simulink model "TVC_Rocket"  (R2026a)
settings: Solver=VariableStepAuto  StopTime=120
values from neighbouring files (symbols this model uses):
  Iyy = 0.0153455729167    [TVC_results_baseline.mat]
  Kp = 5    [TVC_results_baseline.mat]
  L = 0.55    [TVC_results_baseline.mat]
  servo_max = 15    [TVC_results_baseline.mat]
  servo_min = -15    [TVC_results_baseline.mat]
libraries: slpidlib x2
settings Model: Creator=haquangchuong  LastModifiedBy=haquangchuong

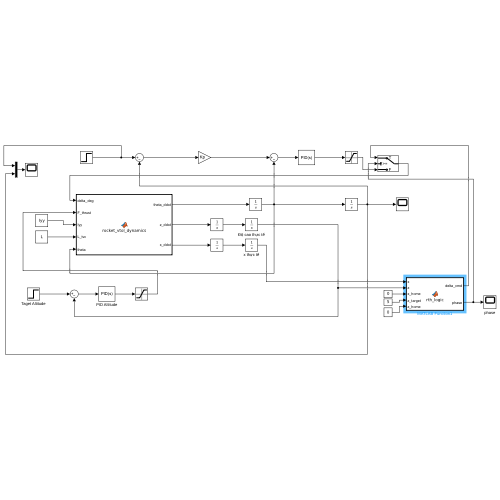
[thumbnail: Simulink's stored preview of the top-level diagram]
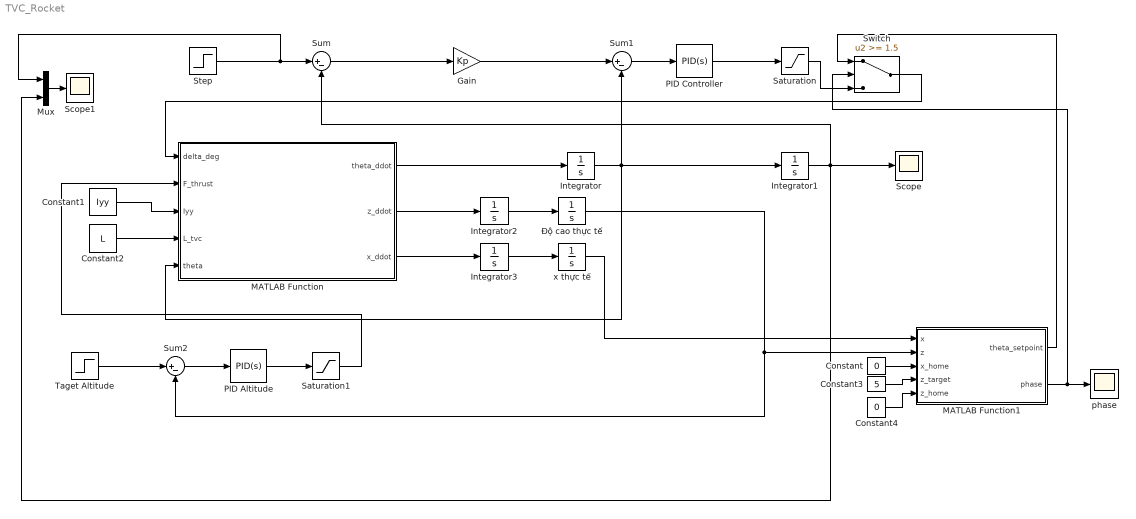
== system TVC_Rocket ==
  Constant : Constant  Value=0
  Constant1 : Constant  Value=Iyy
  Constant2 : Constant  Value=L
  Constant3 : Constant  Value=5
  Constant4 : Constant  Value=0
  Gain : Gain  Gain=Kp
  Integrator{,1..3} (4 alike) : Integrator
  MATLAB Function : MATLAB Function  TreatAsAtomicUnit=on
  MATLAB Function1 : MATLAB Function  TreatAsAtomicUnit=on
  Mux : Mux  Inputs=2
  PID Altitude : slpidlib/PID Controller  Controller=PID  Form=Parallel  TimeDomain=Continuous-time  UseExternalTs=off  SampleTime=-1  IntegratorMethod=Forward Euler  FilterMethod=Forward Euler  ControllerParametersSource=internal  P=2.0  I=0.005  UseKiTs=off  D=1.0  UseExternalDerivativeSource=off  N=100  UseFilter=on  TunerSelectOption=Transfer Function Based (PID Tuner App)  InitialConditionSource=internal  InitialConditionForIntegrator=0  InitialConditionForFilter=0  DifferentiatorICPrevScaledInput=0  ExternalReset=none  TrackingMode=off  Kt=1  LimitOutput=off  SatLimitsSource=internal  UpperSaturationLimit=inf  LowerSaturationLimit=-inf  LinearizeAsGain=on  AntiWindupMode=none  Kb=1  LimitIntegrator=off  UpperIntegratorSaturationLimit=inf  LowerIntegratorSaturationLimit=-inf  POutMin=[]  POutMax=[]  IOutMin=[]  IOutMax=[]  DOutMin=[]  DOutMax=[]  NOutMin=[]  NOutMax=[]  SumOutMin=[]  SumOutMax=[]  SaturationOutMin=[]  SaturationOutMax=[]  PParamMin=[]  PParamMax=[]  IParamMin=[]  IParamMax=[]  DParamMin=[]  DParamMax=[]  NParamMin=[]  NParamMax=[]  KbParamMin=[]  KbParamMax=[]  KtParamMin=[]  KtParamMax=[]  KbOutMin=[]  KbOutMax=[]  KtOutMin=[]  KtOutMax=[]  IntegratorOutMin=[]  IntegratorOutMax=[]  FilterOutMin=[]  FilterOutMax=[]  SumI1OutMin=[]  SumI1OutMax=[]  SumI2OutMin=[]  SumI2OutMax=[]  SumI3OutMin=[]  SumI3OutMax=[]  SumI4OutMin=[]  SumI4OutMax=[]  SumDOutMin=[]  SumDOutMax=[]  DifferentiatorOutMin=[]  DifferentiatorOutMax=[]  FilterDiffOutCoefMin=[]  FilterDiffOutCoefMax=[]  ReciprocalOutMin=[]  ReciprocalOutMax=[]  SumDenOutMin=[]  SumDenOutMax=[]  SumNumOutMin=[]  SumNumOutMax=[]  DivideOutMin=[]  DivideOutMax=[]  UdiffTsProdOutMin=[]  UdiffTsProdOutMax=[]  NTsProdOutMin=[]  NTsProdOutMax=[]  UintegralTsProdOutMin=[]  UintegralTsProdOutMax=[]  UngainTsProdOutMin=[]  UngainTsProdOutMax=[]  ClampingZeroOutDataTypeStr=Inherit: Inherit via back propagation  ClampingZeroOutMin=[]  ClampingZeroOutMax=[]  FilterDenConstantOutDataTypeStr=Inherit: Inherit via back propagation  FilterDenConstantOutMin=[]  FilterDenConstantOutMax=[]  PCopyOutDataTypeStr=Inherit: Inherit via back propagation  PCopyOutMin=[]  PCopyOutMax=[]  NCopyOutDataTypeStr=Inherit: Inherit via back propagation  NCopyOutMin=[]  NCopyOutMax=[]  IntegratorContinuousStateAttributes=''  IntegratorStateMustResolveToSignalObject=off  IntegratorRTWStateStorageClass=Auto  FilterContinuousStateAttributes=''  FilterStateMustResolveToSignalObject=off  FilterRTWStateStorageClass=Auto  ParallelPVariant=InternalParameters  IdealPVariant=Disabled  IVariant=InternalParameters  DVariant=InternalParameters  IntegratorVariant=Continuous  SatVariant=Disabled  AWVariant=Passthrough  PCopyVariant=Disabled  TRVariant=Disabled  FdbkBlocksVariant=Forward  IdealPFdbkVariant=Disabled  SatFdbkVariant=Disabled  DerivativeFilterVariant=ContFilter  NVariant=InternalParameters  NCopyVariant=Disabled  FilterICVariant=InternalICsFilter  IntegratorICVariant=InternalICs  ExternalResetVariant=Disabled  TRSumVariant=Passthrough  SumFdbkVariant=Disabled  SumVariant=Sum_PID  TsampFilterVariant=InternalTs  TsampNgainVariant=Passthrough  TsampIntegralVariant=Disabled_SignalSpec  ExternalSaturationOutDataTypeStr=Inherit: Same as second input  DerivativeSourceVariant=ErrorSignal  PreIntVariant=InternalPreInt
  PID Controller : slpidlib/PID Controller  Controller=PID  Form=Parallel  TimeDomain=Continuous-time  UseExternalTs=off  SampleTime=-1  IntegratorMethod=Forward Euler  FilterMethod=Forward Euler  ControllerParametersSource=internal  P=1.5  I=0.01  UseKiTs=off  D=0.8  UseExternalDerivativeSource=off  N=100  UseFilter=on  TunerSelectOption=Transfer Function Based (PID Tuner App)  InitialConditionSource=internal  InitialConditionForIntegrator=0  InitialConditionForFilter=0  DifferentiatorICPrevScaledInput=0  ExternalReset=none  TrackingMode=off  Kt=1  LimitOutput=off  SatLimitsSource=internal  UpperSaturationLimit=inf  LowerSaturationLimit=-inf  LinearizeAsGain=on  AntiWindupMode=none  Kb=1  LimitIntegrator=off  UpperIntegratorSaturationLimit=inf  LowerIntegratorSaturationLimit=-inf  POutMin=[]  POutMax=[]  IOutMin=[]  IOutMax=[]  DOutMin=[]  DOutMax=[]  NOutMin=[]  NOutMax=[]  SumOutMin=[]  SumOutMax=[]  SaturationOutMin=[]  SaturationOutMax=[]  PParamMin=[]  PParamMax=[]  IParamMin=[]  IParamMax=[]  DParamMin=[]  DParamMax=[]  NParamMin=[]  NParamMax=[]  KbParamMin=[]  KbParamMax=[]  KtParamMin=[]  KtParamMax=[]  KbOutMin=[]  KbOutMax=[]  KtOutMin=[]  KtOutMax=[]  IntegratorOutMin=[]  IntegratorOutMax=[]  FilterOutMin=[]  FilterOutMax=[]  SumI1OutMin=[]  SumI1OutMax=[]  SumI2OutMin=[]  SumI2OutMax=[]  SumI3OutMin=[]  SumI3OutMax=[]  SumI4OutMin=[]  SumI4OutMax=[]  SumDOutMin=[]  SumDOutMax=[]  DifferentiatorOutMin=[]  DifferentiatorOutMax=[]  FilterDiffOutCoefMin=[]  FilterDiffOutCoefMax=[]  ReciprocalOutMin=[]  ReciprocalOutMax=[]  SumDenOutMin=[]  SumDenOutMax=[]  SumNumOutMin=[]  SumNumOutMax=[]  DivideOutMin=[]  DivideOutMax=[]  UdiffTsProdOutMin=[]  UdiffTsProdOutMax=[]  NTsProdOutMin=[]  NTsProdOutMax=[]  UintegralTsProdOutMin=[]  UintegralTsProdOutMax=[]  UngainTsProdOutMin=[]  UngainTsProdOutMax=[]  ClampingZeroOutDataTypeStr=Inherit: Inherit via back propagation  ClampingZeroOutMin=[]  ClampingZeroOutMax=[]  FilterDenConstantOutDataTypeStr=Inherit: Inherit via back propagation  FilterDenConstantOutMin=[]  FilterDenConstantOutMax=[]  PCopyOutDataTypeStr=Inherit: Inherit via back propagation  PCopyOutMin=[]  PCopyOutMax=[]  NCopyOutDataTypeStr=Inherit: Inherit via back propagation  NCopyOutMin=[]  NCopyOutMax=[]  IntegratorContinuousStateAttributes=''  IntegratorStateMustResolveToSignalObject=off  IntegratorRTWStateStorageClass=Auto  FilterContinuousStateAttributes=''  FilterStateMustResolveToSignalObject=off  FilterRTWStateStorageClass=Auto  ParallelPVariant=InternalParameters  IdealPVariant=Disabled  IVariant=InternalParameters  DVariant=InternalParameters  IntegratorVariant=Continuous  SatVariant=Disabled  AWVariant=Passthrough  PCopyVariant=Disabled  TRVariant=Disabled  FdbkBlocksVariant=Forward  IdealPFdbkVariant=Disabled  SatFdbkVariant=Disabled  DerivativeFilterVariant=ContFilter  NVariant=InternalParameters  NCopyVariant=Disabled  FilterICVariant=InternalICsFilter  IntegratorICVariant=InternalICs  ExternalResetVariant=Disabled  TRSumVariant=Passthrough  SumFdbkVariant=Disabled  SumVariant=Sum_PID  TsampFilterVariant=InternalTs  TsampNgainVariant=Passthrough  TsampIntegralVariant=Disabled_SignalSpec  ExternalSaturationOutDataTypeStr=Inherit: Same as second input  DerivativeSourceVariant=ErrorSignal  PreIntVariant=InternalPreInt
  Saturation : Saturate  UpperLimit=servo_max  LowerLimit=servo_min
  Saturation1 : Saturate
  Scope : Scope
      settings: ActiveDisplayYMinimum=-17.498185501340227  ActiveDisplayYMaximum=33.688920146330474
  Scope1 : Scope
      settings: ActiveDisplayYMinimum=-24.629671533739579  ActiveDisplayYMaximum=40.871041025678686
  Step : Step  FinalValue=5  SampleTime=0
  Sum : Sum  Inputs=|+-
  Sum1 : Sum  Inputs=|+-
  Sum2 : Sum  Inputs=|+-
  Switch : Switch  Threshold=1.5  SaturateOnIntegerOverflow=off  InputSameDT=off
  Taget Altitude : Step  FinalValue=5  SampleTime=0
  phase : Scope
      settings: ActiveDisplayYMinimum=1.2513737905524991  ActiveDisplayYMaximum=3.346104044701578  DataLoggingVariableName=ScopeData2
  x thực tế : Integrator
  Độ cao thực tế : Integrator
  wires:
  MATLAB Function/1(theta_ddot) -> Integrator/1
  Integrator/1 -> MATLAB Function/5(theta), Integrator1/1, Sum1/2
  Constant1/1 -> MATLAB Function/3(Iyy)
  Constant2/1 -> MATLAB Function/4(L_tvc)
  Step/1 -> Mux/1, Sum/1
  Integrator1/1 -> Mux/2, Scope/1, Sum/2
  Sum/1 -> Gain/1
  Gain/1 -> Sum1/1
  Sum1/1 -> PID Controller/1
  PID Controller/1 -> Saturation/1
  Mux/1 -> Scope1/1
  MATLAB Function/2(z_ddot) -> Integrator2/1
  Integrator2/1 -> Độ cao thực tế/1
  Taget Altitude/1 -> Sum2/1
  Độ cao thực tế/1 -> MATLAB Function1/2(z), Sum2/2
  Sum2/1 -> PID Altitude/1
  PID Altitude/1 -> Saturation1/1
  Saturation1/1 -> MATLAB Function/2(F_thrust)
  MATLAB Function/3(x_ddot) -> Integrator3/1
  Integrator3/1 -> x thực tế/1
  Constant/1 -> MATLAB Function1/3(x_home)
  Constant3/1 -> MATLAB Function1/4(z_target)
  Constant4/1 -> MATLAB Function1/5(z_home)
  x thực tế/1 -> MATLAB Function1/1(x)
  MATLAB Function1/2(phase) -> phase/1, Switch/2
  Switch/1 -> MATLAB Function/1(delta_deg)
  Saturation/1 -> Switch/3
  MATLAB Function1/1(theta_setpoint) -> Switch/1

== matlab function TVC_Rocket/MATLAB Function1 ==
  data: x input; theta_setpoint output; z input; x_home input; z_target input; z_home input; phase output
function [theta_setpoint, phase] = rth_logic(x, z, x_home, z_target, z_home)
    altitude = -z;
    x_error = x_home - x;

    if altitude < z_target - 0.5
        phase = 1;
        theta_setpoint = 0;

    elseif abs(x_error) > 0.3
        phase = 2;
        % Nghiêng nhẹ để bay ngang — max 3 độ
        theta_setpoint = max(min(0.5 * x_error, 3), -3);

    elseif altitude > 0.1
        phase = 3;
        theta_setpoint = 0;

    else
        phase = 4;
        theta_setpoint = 0;
    end
end

== matlab function TVC_Rocket/MATLAB Function ==
  data: delta_deg input; theta_ddot output; F_thrust input; Iyy input; L_tvc input; theta input; z_ddot output; x_ddot output
function [theta_ddot, z_ddot, x_ddot] = rocket_vtol_dynamics(delta_deg, F_thrust, Iyy, L_tvc, theta)
    m = 0.605;
    g = 9.81;
    delta_rad = deg2rad(delta_deg);
    theta_rad = deg2rad(theta);

    % Trục Pitch
    torque = F_thrust * sin(delta_rad) * L_tvc ...
           - m * g * (L_tvc * 0.5) * sin(theta_rad);
    theta_ddot = torque / Iyy;

    % Trục Z (Cao độ)
    F_vertical = F_thrust * cos(delta_rad + theta_rad);
    z_ddot = (F_vertical - m*g) / m;

    % Trục X (Ngang — RTH cần cái này)
    F_horizontal = F_thrust * sin(delta_rad + theta_rad);
    x_ddot = F_horizontal / m;
end
